simulink model "ExperimentModelPIDFeedFowardDigital"  (R2020b)
settings: Solver=FixedStepDiscrete  StartTime=0.0  StopTime=10  FixedStep=Ts  RelTol=1e-3
undefined symbols (not defined in the file): Beq, CDer, CInt, DiscIntNeverNeededParam, drv, gbox, Jeq, Kd, Ki, Kp, Kw, mld, mot, National_Instruments, PCI, Req, rpm2degs, rpm2rads, sens, Ts
libraries: sldrtlib x3, simulink x1
settings Model: ExtModeTrigDuration=100000  Creator=umbe  LastModifiedBy=Diego
settings DataIOCC: ReturnWorkspaceOutputs=off
settings RTWCC: Description=Simulink Desktop Real-Time  SystemTargetFile=sldrt.tlc  TemplateMakefile=sldrt.tmf  RTWCompilerOptimization=on
settings CodeAppCC: MaxIdLength=95
settings SimulinkDesktopRealTimeCC: TargetPreCompLibLocation=C:\Program Files\MATLAB\R2020b\toolbox\sldrt\lib\win64

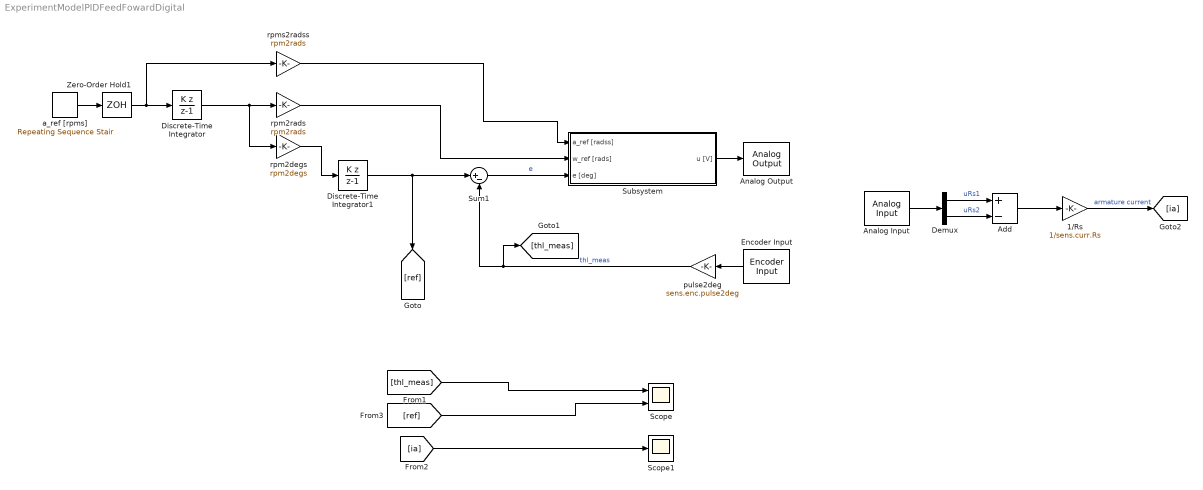
== system ExperimentModelPIDFeedFowardDigital ==
  1/Rs : Gain  Gain=1/sens.curr.Rs
  Add : Sum  Inputs=+-
  Analog Input : sldrtlib/Analog Input  SampleTime=Ts  MaxMissedTicks=10  ShowMissedTicks=off  YieldWhenWaiting=off  DrvName=National_Instruments/PCI-6221  DrvAddress=4294967295  DrvOptions=[0 0 0 2 0]  Channels=[1 2]  RangeMode=1  VoltRange=1  DataType=1
      settings: AttributesFormatString=National Instruments\nPCI-6221 [auto]
  Analog Output : sldrtlib/Analog Output  SampleTime=Ts  MaxMissedTicks=10  ShowMissedTicks=off  YieldWhenWaiting=off  DrvName=National_Instruments/PCI-6221  DrvAddress=4294967295  DrvOptions=[0 0 0 2 0]  Channels=1  RangeMode=1  VoltRange=1  InitialValue=0  FinalValue=0
      settings: AttributesFormatString=National Instruments\nPCI-6221 [auto]
  Demux : Demux  Outputs=2
  Discrete-Time Integrator : DiscreteIntegrator  IntegratorMethod=Accumulation: Backward Euler  gainval=Ts  SampleTime=Ts  ICPrevOutput=DiscIntNeverNeededParam  ICPrevScaledInput=DiscIntNeverNeededParam
  Discrete-Time Integrator1 : DiscreteIntegrator  IntegratorMethod=Accumulation: Backward Euler  gainval=Ts  SampleTime=Ts  ICPrevOutput=DiscIntNeverNeededParam  ICPrevScaledInput=DiscIntNeverNeededParam
  Encoder Input : sldrtlib/Encoder Input  SampleTime=Ts  MaxMissedTicks=10  ShowMissedTicks=off  YieldWhenWaiting=off  DrvName=National_Instruments/PCI-6221  DrvAddress=4294967295  DrvOptions=[0 0 0 2 0]  Channels=1  QuadMode=3  IndexPulse=1  InputFilter=Inf  DataType=1
      settings: AttributesFormatString=National Instruments\nPCI-6221 [auto]
  Scope : Scope  NumInputPorts=2
  Scope1 : Scope
  Subsystem : Subsystem
  Sum1 : Sum  Inputs=|+-
  Zero-Order Hold1 : ZeroOrderHold  SampleTime=Ts
  a_ref [rpms] : simulink/Sources/Repeating Sequence Stair  OutValues=[900 0 -900 -900 0 900].'  tsamp=0.5  OutMin=[]  OutMax=[]  OutDataTypeStr=double  OutputDataTypeScalingMode=double  OutDataType=fixdt(0,8)  ConRadixGroup=Best Precision: Vector-wise  OutScaling=2^-12
  pulse2deg : Gain  Gain=sens.enc.pulse2deg
  rpm2degs : Gain  Gain=rpm2degs
  rpm2rads : Gain  Gain=rpm2rads
  rpms2radss : Gain  Gain=rpm2rads
  wires:
  1/Rs/1 -> [ia]  "armature current"
  Add/1 -> 1/Rs/1
  Demux/1 -> Add/1  "uRs1"
  Demux/2 -> Add/2  "uRs2"
  pulse2deg/1 -> [thl_meas], Sum1/2  "thl_meas"
  Sum1/1 -> Subsystem/3(e [deg])  "e"
  [thl_meas] -> Scope/1
  [ia] -> Scope1/1
  Encoder Input/1 -> pulse2deg/1
  Analog Input/1 -> Demux/1
  Subsystem/1(u [V]) -> Analog Output/1
  Discrete-Time Integrator1/1 -> Sum1/1, [ref]
  [ref] -> Scope/2
  Zero-Order Hold1/1 -> rpms2radss/1, Discrete-Time Integrator/1
  Discrete-Time Integrator/1 -> rpm2rads/1, rpm2degs/1
  a_ref [rpms]/1 -> Zero-Order Hold1/1
  rpm2degs/1 -> Discrete-Time Integrator1/1
  rpm2rads/1 -> Subsystem/2(w_ref [rads])
  rpms2radss/1 -> Subsystem/1(a_ref [radss])

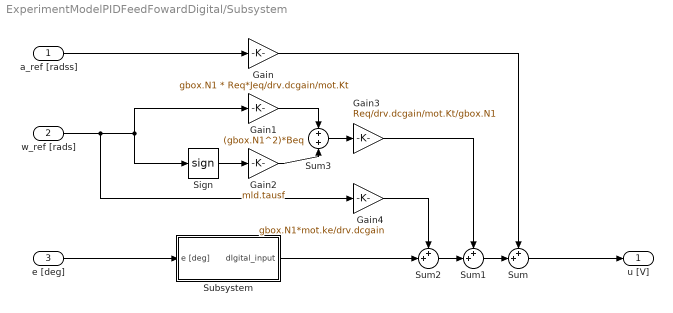
== system ExperimentModelPIDFeedFowardDigital/Subsystem ==
  a_ref [radss] : Inport
  w_ref [rads] : Inport  Port=2
  e [deg] : Inport  Port=3
  Gain : Gain  Gain=gbox.N1 * Req*Jeq/drv.dcgain/mot.Kt
  Gain1 : Gain  Gain=(gbox.N1^2)*Beq
  Gain2 : Gain  Gain=mld.tausf
  Gain3 : Gain  Gain=Req/drv.dcgain/mot.Kt/gbox.N1
  Gain4 : Gain  Gain=gbox.N1*mot.ke/drv.dcgain
  Sign : Signum
  Subsystem : Subsystem
  Sum : Sum  Inputs=++|
  Sum1 : Sum  Inputs=++|
  Sum2 : Sum  Inputs=++|
  Sum3 : Sum  Inputs=+|+
  u [V] : Outport
  wires:
  e [deg]/1 -> Subsystem/1(e [deg])
  a_ref [radss]/1 -> Gain/1
  Sum/1 -> u [V]/1
  Gain/1 -> Sum/1
  w_ref [rads]/1 -> Gain1/1, Sign/1, Gain4/1
  Sign/1 -> Gain2/1
  Subsystem/1(dIgital_input) -> Sum2/2
  Sum3/1 -> Gain3/1
  Gain2/1 -> Sum3/2
  Gain1/1 -> Sum3/1
  Gain3/1 -> Sum1/1
  Sum1/1 -> Sum/2
  Gain4/1 -> Sum2/1
  Sum2/1 -> Sum1/2

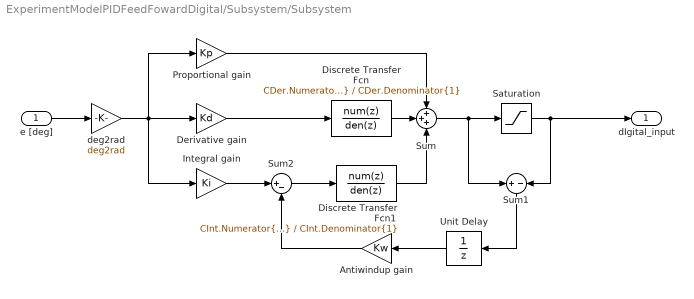
== system ExperimentModelPIDFeedFowardDigital/Subsystem/Subsystem ==
  e [deg] : Inport
  Antiwindup gain : Gain  Gain=Kw
  Derivative gain : Gain  Gain=Kd
  Discrete Transfer Fcn : DiscreteTransferFcn  Numerator=CDer.Numerator{1}  Denominator=CDer.Denominator{1}  SampleTime=Ts
  Discrete Transfer Fcn1 : DiscreteTransferFcn  Numerator=CInt.Numerator{1}  Denominator=CInt.Denominator{1}  SampleTime=Ts
  Integral gain : Gain  Gain=Ki
  Proportional gain : Gain  Gain=Kp
  Saturation : Saturate  UpperLimit=10  LowerLimit=-10
  Sum : Sum  Inputs=+++
  Sum1 : Sum  Inputs=+|-
  Sum2 : Sum  Inputs=|+-
  Unit Delay : UnitDelay  SampleTime=-1  HasFrameUpgradeWarning=on
  deg2rad : Gain  Gain=deg2rad
  dIgital_input : Outport
  wires:
  Proportional gain/1 -> Sum/1
  Discrete Transfer Fcn/1 -> Sum/2
  Derivative gain/1 -> Discrete Transfer Fcn/1
  Discrete Transfer Fcn1/1 -> Sum/3
  deg2rad/1 -> Proportional gain/1, Derivative gain/1, Integral gain/1
  e [deg]/1 -> deg2rad/1
  Antiwindup gain/1 -> Sum2/2
  Sum1/1 -> Unit Delay/1
  Saturation/1 -> Sum1/2, dIgital_input/1
  Sum/1 -> Saturation/1, Sum1/1
  Integral gain/1 -> Sum2/1
  Sum2/1 -> Discrete Transfer Fcn1/1
  Unit Delay/1 -> Antiwindup gain/1
